simulink model "farrow_interpolator"  (R2016a)
settings: Solver=VariableStepAuto  StartTime=0.0  StopTime=10.0  RelTol=1e-3
settings Model: Creator=coltmt  LastModifiedBy=coltmt

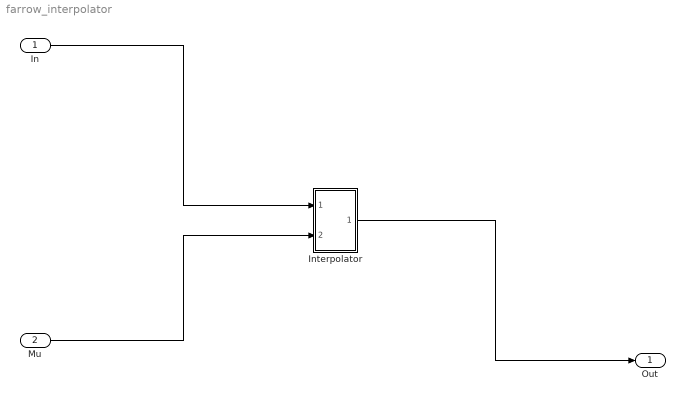
== system farrow_interpolator ==
  In : Inport
  "Mu " : Inport  Port=2
  "Interpolator " : Subsystem
  "Out " : Outport
  wires:
  In/1 -> "Interpolator "/1(In1)
  "Mu "/1 -> "Interpolator "/2(In2)
  "Interpolator "/1(Out1) -> "Out "/1

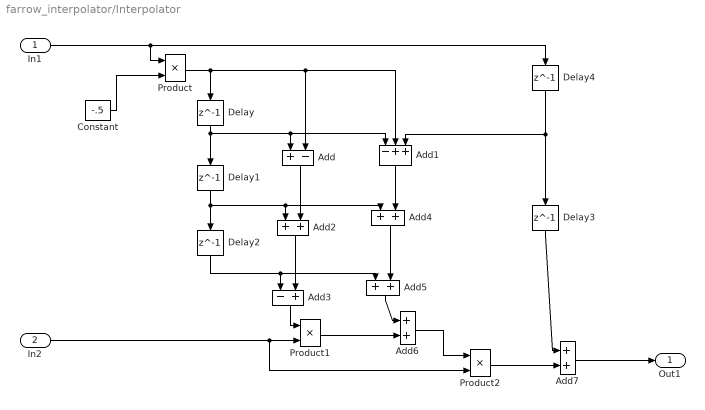
== system farrow_interpolator/Interpolator  ==
  In1 : Inport
  In2 : Inport  Port=2
  Add : Sum  Inputs=+-
  Add1 : Sum  Inputs=-++
  Add{2,4..7} (5 alike) : Sum
  Add3 : Sum  Inputs=-+
  Constant : Constant  Value=-.5
  Delay{,1..4} (5 alike) : Delay  DelayLength=1  InputProcessing=Columns as channels (frame based)
  Product : Product
  Product1 : Product
  Product2 : Product
  Out1 : Outport
  wires:
  In1/1 -> Delay4/1, Product/1
  Constant/1 -> Product/2
  Add3/1 -> Product1/1
  Delay/1 -> Delay1/1, Add1/1, Add/1
  Delay2/1 -> Add5/1, Add3/1
  Add6/1 -> Product2/1
  Product/1 -> Add1/2, Add/2, Delay/1
  Delay4/1 -> Add1/3, Delay3/1
  Add5/1 -> Add6/1
  Add7/1 -> Out1/1
  Product2/1 -> Add7/2
  Add2/1 -> Add3/2
  Add1/1 -> Add4/2
  Add/1 -> Add2/2
  Product1/1 -> Add6/2
  Delay3/1 -> Add7/1
  Add4/1 -> Add5/2
  In2/1 -> Product2/2, Product1/2
  Delay1/1 -> Add4/1, Add2/1, Delay2/1
